simulink model "IM_model"  (R2022b)
settings: Solver=ode23s  StartTime=0.0  StopTime=0.8  MaxStep=1e-3  RelTol=1e-3  EnableMultiTasking=on
values from neighbouring files (symbols this model uses):
  B = 0.068    [IM_model_parameters.m]
  J = 0.4    [IM_model_parameters.m]
  Lks = Ls- Lm^2/Lr    (= 0.00442538071066)    [IM_model_parameters.m]
  Lm = 57e-3    (= 0.057)    [IM_model_parameters.m]
  np = 3    [IM_model_parameters.m]
  Rr = 0.175    [IM_model_parameters.m]
  Rs = 0.24    [IM_model_parameters.m]
undefined symbols (not defined in the file or in its folder): j
Description:
  | Mattia Rossi
settings Model: PacingRate=0.001000  Creator=matti  LastModifiedBy=benve
settings SolverCC: AlgebraicLoopSolver=TrustRegion
settings DataIOCC: LimitDataPoints=on  SaveFormat=Array  ReturnWorkspaceOutputs=off
settings OptimizationCC: LifeSpan=inf
settings DebuggingCC: SolverPrmCheckMsg=warning  UnconnectedInputMsg=warning  UnconnectedOutputMsg=warning  UnconnectedLineMsg=warning  SFUnexpectedBacktrackingDiag=warning  SFNoUnconditionalDefaultTransitionDiag=warning  SFExecutionAtInitializationDiag=none  SFMachineParentedDataDiag=warning  ArithmeticOperatorsInVariantConditions=warning
settings HardwareCC: ProdBitPerPointer=32  ProdBitPerSizeT=32  ProdBitPerPtrDiffT=32  ProdLargestAtomicFloat=None  ProdIntDivRoundTo=Undefined  ProdEndianess=Unspecified  ProdWordSize=32  ProdHWDeviceType=32-bit Generic
settings ModelReferenceCC: EnableRefExpFcnMdlSchedulingChecks=on  PropagateSignalLabelsOutOfModel=off
settings SFSimCC: SimUseLocalCustomCode=off  CustomCodeUndefinedFunction=UseInterfaceOnly
settings RTWCC: RTWUseLocalCustomCode=off
settings CodeAppCC: StateflowObjectComments=on
settings GRTTargetCC: TargetLangStandard=C89/C90 (ANSI)
settings ConfigComp: CovMetricSettings=dw  CovSaveCumulativeToWorkspaceVar=on  CovSaveSingleToWorkspaceVar=on  CovExternalEMLEnable=off  CovSFcnEnable=off

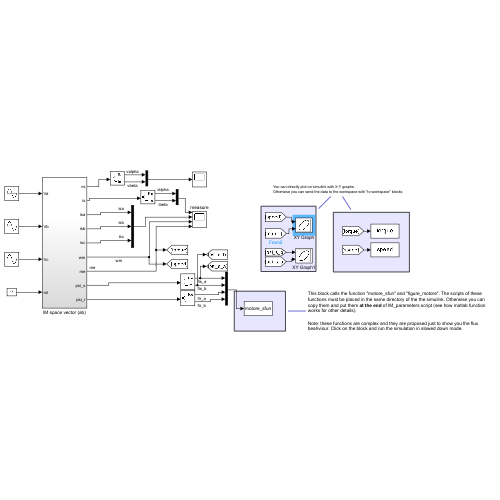
[thumbnail: Simulink's stored preview of the top-level diagram]
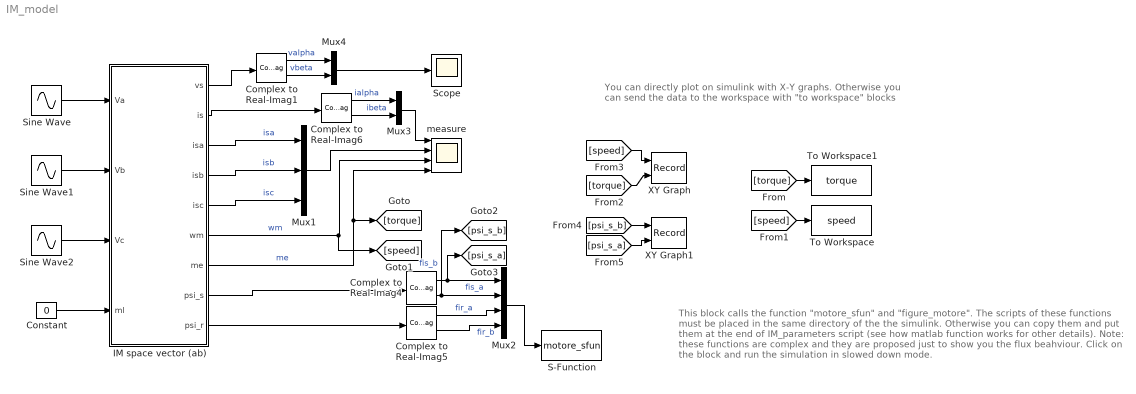
== system IM_model ==
  note: This block calls the function "motore_sfun" and "figure_motore". The scripts of these functions must be placed in the same directory of the the simulink. Otherwise you can copy them and put them at the end of IM_parameters script (see how matlab function works for other details).
      |
      | Note: these functions are complex and they are proposed just to show you the flux beahviour. Click on the block and run the simulation in slowed down mode.
  note: You can directly plot on simulink with X-Y graphs.
      | Otherwise you can send the data to the workspace with "to workspace" blocks
  Complex to Real-Imag{1,4..6} (4 alike) : ComplexToRealImag
  Constant : Constant  Value=0
  IM space vector (ab) : Subsystem
  Mux1 : Mux  Inputs=3
  Mux2 : Mux
  Mux3 : Mux  Inputs=2
  Mux4 : Mux  Inputs=2
  S-Function : S-Function  FunctionName=motore_sfun  SFunctionDeploymentMode=off  EnableBusSupport=off
      settings: OpenFcn=figure_motore
  Scope : Scope
  Sine Wave : Sin  Amplitude=380*sqrt(2)  Frequency=2*pi*50  SampleTime=0
  Sine Wave1 : Sin  Amplitude=380*sqrt(2)  Frequency=2*pi*50  Phase=-2*pi/3  SampleTime=0
  Sine Wave2 : Sin  Amplitude=380*sqrt(2)  Frequency=2*pi*50  Phase=-4*pi/3  SampleTime=0
  To Workspace : ToWorkspace  VariableName=speed  SampleTime=-1
  To Workspace1 : ToWorkspace  VariableName=torque  SampleTime=-1
  XY Graph : Record  FileSettingsInternal="{\"entries\":[{\"content\":{\"excelSettings\":{\"content\":{},\"type\":\"Streamout.ExcelSettings\"}},\"type\":\"Streamout.FileSettingStorage\",\"uuid\":\"4af16882-2086-40a6-94ab-f8150837ffa8\"}],\"packageUris\":[\"http://schema.mathworks.com/mf0/streamout_blocks/R2020a\"],\"version\":\"1.0\"}"  Layout=[1 1]  SignalsInternal="{\"entries\":[{\"content\":{\"signals\":[{\"content\":{\"blockPath\":[\"IM_model/XY Graph\"],\"channel\":[],\"dimensions\":[1],\"domain\":\"IM_model/XY Graph\",\"lineColor\":\"#a2142f\",\"plots\":[1],\"port\":1,\"sid\":[\"\"],\"signalID\":2525,\"signalName\":\"From3\"},\"type\":\"RecordBlkView.Signal\",\"uuid\":\"a5c80903-c1c6-48d7-9634-96254d246ccd\"},{\"content\":{\"blockPath\":[\"IM_model/XY Graph\"],\"channel\":[],\"dimensions\":[1],\"domain\":\"IM_model/XY Graph\",\"lineColor\":\"#139fff\",\"plots\":[1],\"port\":2,\"sid\":[\"\"],\"signalID\":2529,\"signalName\":\"From2\"},\"type\":\"RecordBlkView.Signal\",\"uuid\":\"70254788-b274-4115-bf2d-0a6052768582\"}]},\"type\":\"RecordBlkView.InputSignals\",\"uuid\":\"a9c73759-3092-44e1-8a36-f1f6f6828635\"}],\"packageUris\":[\"http://schema.mathworks.com/mf0/streamout_blocks/R2020a\"],\"version\":\"1.0\"}"  VisualizationBindings="{\"xyplotplugin\":{\"info\":[{\"series\":[{\"bindingParametersList\":[{\"parameter\":\"X-Axis\",\"signalID\":2525,\"signalName\":\"From3\"},{\"parameter\":\"Y-Axis\",\"signalID\":2529,\"signalName\":\"From2\"}],\"seriesID\":51756}],\"subplotID\":1}]}}"  CompatibilityTag=XY
  XY Graph1 : Record  FileSettingsInternal="{\"entries\":[{\"content\":{\"excelSettings\":{\"content\":{},\"type\":\"Streamout.ExcelSettings\"}},\"type\":\"Streamout.FileSettingStorage\",\"uuid\":\"43a2d26a-f79d-41d1-ad3e-8586555017c5\"}],\"packageUris\":[\"http://schema.mathworks.com/mf0/streamout_blocks/R2020a\"],\"version\":\"1.0\"}"  Layout=[1 1]  SignalsInternal="{\"entries\":[{\"content\":{\"signals\":[{\"content\":{\"blockPath\":[\"IM_model/XY Graph1\"],\"channel\":[],\"dimensions\":[1],\"domain\":\"IM_model/XY Graph1\",\"lineColor\":\"#a2142f\",\"plots\":[1],\"port\":1,\"sid\":[\"\"],\"signalID\":2533,\"signalName\":\"From4\"},\"type\":\"RecordBlkView.Signal\",\"uuid\":\"26a16e83-51c8-495f-92a0-de0a5ec67a35\"},{\"content\":{\"blockPath\":[\"IM_model/XY Graph1\"],\"channel\":[],\"dimensions\":[1],\"domain\":\"IM_model/XY Graph1\",\"lineColor\":\"#139fff\",\"plots\":[1],\"port\":2,\"sid\":[\"\"],\"signalID\":2537,\"signalName\":\"From5\"},\"type\":\"RecordBlkView.Signal\",\"uuid\":\"ab6ee6ef-c39b-4f87-9cbc-bbb65fed6dd1\"}]},\"type\":\"RecordBlkView.InputSignals\",\"uuid\":\"62ab3ea0-0944-4632-a8da-75c720f91366\"}],\"packageUris\":[\"http://schema.mathworks.com/mf0/streamout_blocks/R2020a\"],\"version\":\"1.0\"}"  VisualizationBindings="{\"xyplotplugin\":{\"info\":[{\"series\":[{\"bindingParametersList\":[{\"parameter\":\"X-Axis\",\"signalID\":2533,\"signalName\":\"From4\"},{\"parameter\":\"Y-Axis\",\"signalID\":2537,\"signalName\":\"From5\"}],\"seriesID\":18533}],\"subplotID\":1}]}}"  CompatibilityTag=XY
  measure : Scope  NumInputPorts=4
  wires:
  Constant/1 -> IM space vector (ab)/4(ml)
  IM space vector (ab)/3(isa) -> Mux1/1  "isa"
  IM space vector (ab)/4(isb) -> Mux1/2  "isb"
  IM space vector (ab)/5(isc) -> Mux1/3  "isc"
  Mux1/1 -> measure/2
  Complex to Real-Imag4/1 -> Mux2/1, [psi_s_a]  "fis_a"
  Complex to Real-Imag4/2 -> [psi_s_b], Mux2/2  "fis_b"
  Complex to Real-Imag5/1 -> Mux2/3  "fir_a"
  Complex to Real-Imag5/2 -> Mux2/4  "fir_b"
  IM space vector (ab)/8(psi_s) -> Complex to Real-Imag4/1
  Sine Wave/1 -> IM space vector (ab)/1(Va)
  Sine Wave1/1 -> IM space vector (ab)/2(Vb)
  Sine Wave2/1 -> IM space vector (ab)/3(Vc)
  Mux2/1 -> S-Function/1
  IM space vector (ab)/2(is) -> Complex to Real-Imag6/1
  Complex to Real-Imag6/1 -> Mux3/1  "ialpha"
  Complex to Real-Imag6/2 -> Mux3/2  "ibeta"
  Mux3/1 -> measure/1
  IM space vector (ab)/6(wm) -> [speed], measure/3  "wm"
  IM space vector (ab)/9(psi_r) -> Complex to Real-Imag5/1
  IM space vector (ab)/7(me) -> [torque], measure/4  "me"
  [torque] -> To Workspace1/1
  [speed] -> To Workspace/1
  Mux4/1 -> Scope/1
  Complex to Real-Imag1/2 -> Mux4/2  "vbeta"
  Complex to Real-Imag1/1 -> Mux4/1  "valpha"
  IM space vector (ab)/1(vs) -> Complex to Real-Imag1/1
  [speed] -> XY Graph/1
  [torque] -> XY Graph/2
  [psi_s_b] -> XY Graph1/1
  [psi_s_a] -> XY Graph1/2

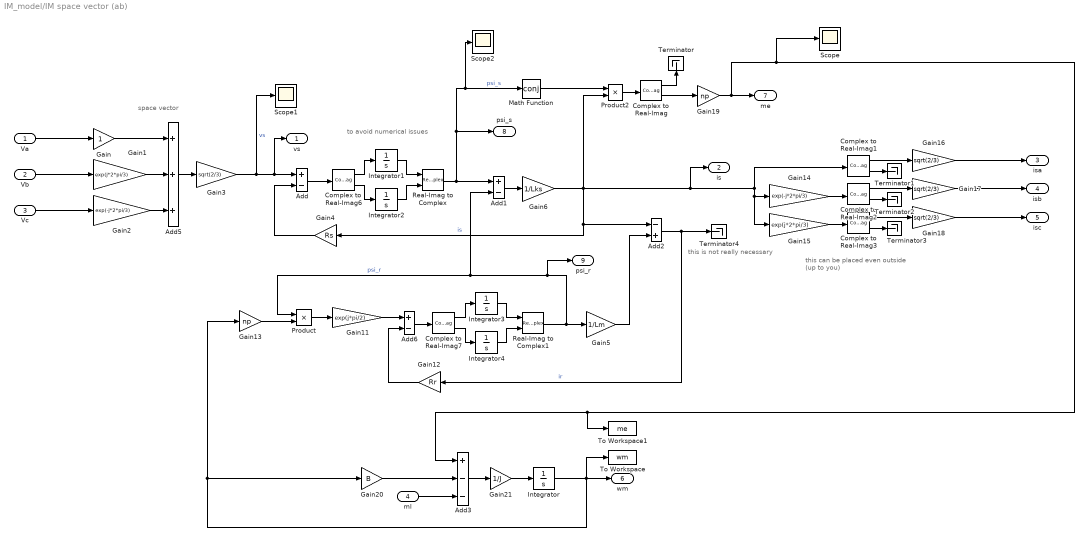
== system IM_model/IM space vector (ab) ==
  note: to avoid numerical issues
  note: this is
      | not really necessary
  note: this can be placed even outside
      | (up to you)
  note: space vector
  Va : Inport
  Vb : Inport  Port=2
  Vc : Inport  Port=3
  ml : Inport  Port=4
  Add : Sum  Inputs=+-
  Add1 : Sum  Inputs=+-
  Add2 : Sum  Inputs=-+
  Add3 : Sum  Inputs=+--
  Add5 : Sum  Inputs=+++
  Add6 : Sum  Inputs=+-
  Complex to Real-Imag{,1..3,6..7} (6 alike) : ComplexToRealImag
  Gain : Gain
  Gain1 : Gain  Gain=exp(j*2*pi/3)
  Gain11 : Gain  Gain=exp(j*pi/2)
  Gain12 : Gain  Gain=Rr
  Gain13 : Gain  Gain=np
  Gain14 : Gain  Gain=exp(-j*2*pi/3)
  Gain15 : Gain  Gain=exp(j*2*pi/3)
  Gain{3,16..18} (4 alike) : Gain  Gain=sqrt(2/3)
  Gain19 : Gain  Gain=np
  Gain2 : Gain  Gain=exp(-j*2*pi/3)
  Gain20 : Gain  Gain=B
  Gain21 : Gain  Gain=1/J
  Gain4 : Gain  Gain=Rs
  Gain5 : Gain  Gain=1/Lm
  Gain6 : Gain  Gain=1/Lks
  Integrator{,1..4} (5 alike) : Integrator
  Math Function : Math  Operator=conj  SignedPower=on
  Product : Product
  Product2 : Product
  Real-Imag to Complex : RealImagToComplex
  Real-Imag to Complex1 : RealImagToComplex
  Scope : Scope
  Scope1 : Scope
  Scope2 : Scope
  Terminator{,1..4} (5 alike) : Terminator
  To Workspace : ToWorkspace  VariableName=wm  SampleTime=-1
  To Workspace1 : ToWorkspace  VariableName=me  SampleTime=-1
  vs : Outport  VectorParamsAs1DForOutWhenUnconnected=off
  is : Outport  Port=2  VectorParamsAs1DForOutWhenUnconnected=off
  isa : Outport  Port=3  VectorParamsAs1DForOutWhenUnconnected=off
  isb : Outport  Port=4  VectorParamsAs1DForOutWhenUnconnected=off
  isc : Outport  Port=5  VectorParamsAs1DForOutWhenUnconnected=off
  wm : Outport  Port=6  VectorParamsAs1DForOutWhenUnconnected=off
  me : Outport  Port=7  VectorParamsAs1DForOutWhenUnconnected=off
  psi_s : Outport  Port=8  VectorParamsAs1DForOutWhenUnconnected=off
  psi_r : Outport  Port=9  VectorParamsAs1DForOutWhenUnconnected=off
  wires:
  Gain5/1 -> Add2/2
  Real-Imag to Complex/1 -> Add1/1, psi_s/1, Scope2/1, Math Function/1  "psi_s"
  Gain6/1 -> Gain4/1, Add2/1, is/1, Gain15/1, Gain14/1, Complex to Real-Imag1/1, Product2/2  "is"
  Gain2/1 -> Add5/3
  Gain/1 -> Add5/1
  Gain1/1 -> Add5/2
  Gain4/1 -> Add/2
  Add1/1 -> Gain6/1
  Real-Imag to Complex1/1 -> Gain5/1, psi_r/1, Add1/2, Product/1  "psi_r"
  Add5/1 -> Gain3/1
  Gain3/1 -> Scope1/1, vs/1, Add/1  "vs"
  Product/1 -> Gain11/1
  Product2/1 -> Complex to Real-Imag/1
  Complex to Real-Imag/1 -> Terminator/1
  Complex to Real-Imag2/2 -> Terminator2/1
  Integrator/1 -> To Workspace/1, wm/1, Gain13/1, Gain20/1
  Complex to Real-Imag/2 -> Gain19/1
  Gain17/1 -> isb/1
  Vb/1 -> Gain1/1
  Va/1 -> Gain/1
  Vc/1 -> Gain2/1
  Gain16/1 -> isa/1
  ml/1 -> Add3/3
  Gain18/1 -> isc/1
  Math Function/1 -> Product2/1
  Add3/1 -> Gain21/1
  Gain13/1 -> Product/2
  Gain20/1 -> Add3/2
  Gain14/1 -> Complex to Real-Imag2/1
  Gain15/1 -> Complex to Real-Imag3/1
  Complex to Real-Imag3/2 -> Terminator3/1
  Complex to Real-Imag1/1 -> Gain16/1
  Gain21/1 -> Integrator/1
  Complex to Real-Imag1/2 -> Terminator1/1
  Complex to Real-Imag3/1 -> Gain18/1
  Complex to Real-Imag2/1 -> Gain17/1
  Gain12/1 -> Add6/2
  Gain11/1 -> Add6/1
  Add/1 -> Complex to Real-Imag6/1
  Integrator2/1 -> Real-Imag to Complex/2
  Integrator1/1 -> Real-Imag to Complex/1
  Complex to Real-Imag6/1 -> Integrator1/1
  Complex to Real-Imag6/2 -> Integrator2/1
  Add6/1 -> Complex to Real-Imag7/1
  Integrator4/1 -> Real-Imag to Complex1/2
  Integrator3/1 -> Real-Imag to Complex1/1
  Complex to Real-Imag7/1 -> Integrator3/1
  Complex to Real-Imag7/2 -> Integrator4/1
  Add2/1 -> Terminator4/1, Gain12/1  "ir"
  Gain19/1 -> Scope/1, To Workspace1/1, Add3/1, me/1
